simulink model "DAB_OL_loss_cal_2023b"  (R2023b)
settings: Solver=VariableStepAuto  StartTime=0.0  StopTime=0.3  RelTol=1e-3
undefined symbols (not defined in the file): Ion, Lithium, powergui, spspowerguiLib
libraries: spsMeanLib x9, spsMosfetLib x8, spsVoltageMeasurementLib x6, spsCurrentMeasurementLib x4, spsSeriesRLCBranchLib x4, eeGeneralControl x4, spsBatteryLib x1, spsDCVoltageSourceLib x1, spsLinearTransformerLib x1, spsRMSLib x1, simulink x1
settings Model: Creator=Project_Account  LastModifiedBy=saivi
settings ModelReferenceCC: EnableRefExpFcnMdlSchedulingChecks=on
settings ConfigComp: CovBoundaryAbsTol=1.0e-5

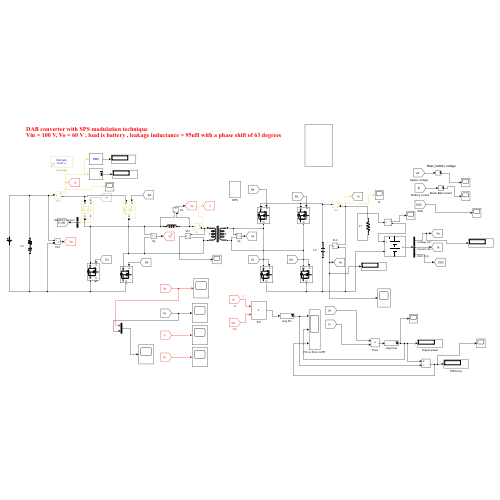
[thumbnail: Simulink's stored preview of the top-level diagram]
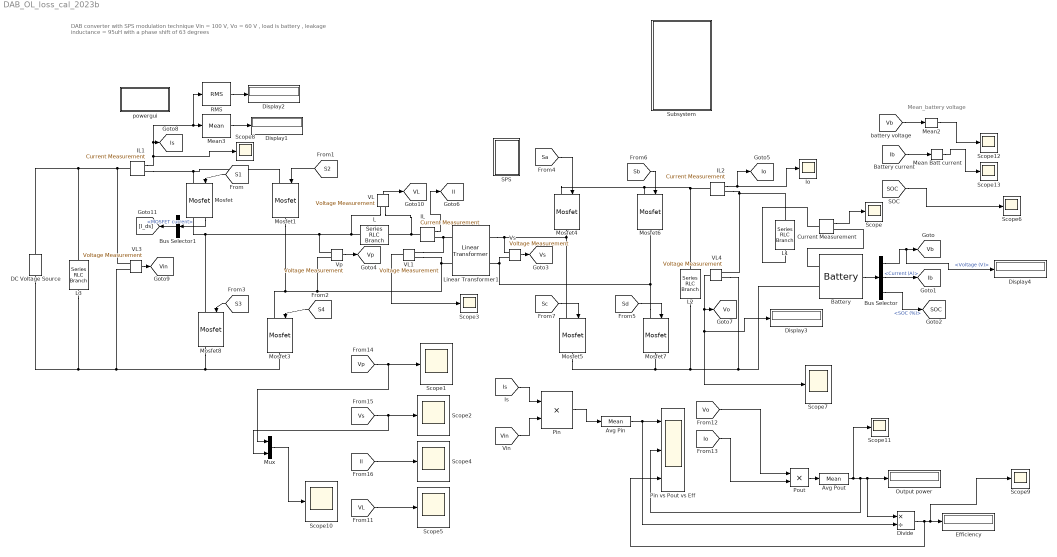
== system DAB_OL_loss_cal_2023b ==
  note: Mean_battery voltage
  note: DAB converter with SPS modulation technique
      | Vin = 100 V, Vo = 60 V , load is battery , leakage inductance = 95uH with a phase shift of 63 degrees
  Avg Pin : spsMeanLib/Mean  Freq=50000  Vinit=0  Ts=1e-7
  Avg Pout : spsMeanLib/Mean  Freq=50000  Vinit=0  Ts=1e-7
  Battery : spsBatteryLib/Battery  BatType=Lithium-Ion  NomV=60  NomQ=120  SOC=60  Batt_Tr=0.1  PresetModel=on  MaxQ=120  MinV=45  FullV=69.8392  Dis_rate=52.1739  R=0.005  Normal_OP=108.5217  expZone="[64.8232      5.89565]"
  Bus Selector : BusSelector  OutputSignals=Voltage (V),Current (A),SOC (%)
  Bus Selector1 : BusSelector  OutputSignals=MOSFET current
  Current Measurement : spsCurrentMeasurementLib/Current Measurement  PhasorSimulation=off  OutputType=Complex  PSBequivalent=0
  DC Voltage Source : spsDCVoltageSourceLib/DC Voltage Source  Amplitude=400  Measurements=None
  Display{1..4} (4 alike) : Display
  Divide : Product  Inputs=*/
  Efficiency : Display
  IL : spsCurrentMeasurementLib/Current Measurement  PhasorSimulation=off  OutputType=Complex  PSBequivalent=0
  IL1 : spsCurrentMeasurementLib/Current Measurement  PhasorSimulation=off  OutputType=Complex  PSBequivalent=0
  IL2 : spsCurrentMeasurementLib/Current Measurement  PhasorSimulation=off  OutputType=Complex  PSBequivalent=0
  Io : Scope
  L : spsSeriesRLCBranchLib/Series RLC Branch  LConnTagsString=__new0  RConnTagsString=__new0  BranchType=L  Resistance=1  Inductance=95e-6  SetiL0=off  InitialCurrent=0  Capacitance=1e-6  Setx0=off  InitialVoltage=0  Measurements=None
  L1 : spsSeriesRLCBranchLib/Series RLC Branch  LConnTagsString=__new0  RConnTagsString=__new0  BranchType=R  Resistance=0.01  Inductance=19.108e-6*2  SetiL0=off  InitialCurrent=0  Capacitance=1000e-6  Setx0=off  InitialVoltage=0  Measurements=None
  L2 : spsSeriesRLCBranchLib/Series RLC Branch  LConnTagsString=__new0  RConnTagsString=__new0  BranchType=C  Resistance=0.8  Inductance=19.108e-6*2  SetiL0=off  InitialCurrent=0  Capacitance=1200e-6  Setx0=off  InitialVoltage=0  Measurements=None
  L3 : spsSeriesRLCBranchLib/Series RLC Branch  LConnTagsString=__new0  RConnTagsString=__new0  BranchType=RC  Resistance=0.8  Inductance=19.108e-6*2  SetiL0=off  InitialCurrent=0  Capacitance=1200e-6  Setx0=off  InitialVoltage=0  Measurements=None
  Linear Transformer1 : spsLinearTransformerLib/Linear Transformer  UNITS=SI  NominalPower=[1500 50000 ]  winding1=[400 0 0]  winding2=[60 0 0]  ThreeWindings=off  winding3=[3.15e+05 0.7938 0.084225]  RmLm=[5000 5866]  Measurements=None  DataType=on
  Mean Batt current : spsMeanLib/Mean  Freq=20000  Vinit=0  Ts=1e-7
  Mean2 : spsMeanLib/Mean  Freq=20000  Vinit=0  Ts=1e-7
  Mean3 : spsMeanLib/Mean  Freq=15000  Vinit=0  Ts=1e-6
  Mosfet : spsMosfetLib/Mosfet  Ron=0.01  Lon=0  Rd=0.01  Vfd=0  IC=0  Rs=1e5  Cs=inf  Measurements=on
  Mosfet{1,3..7} (6 alike) : spsMosfetLib/Mosfet  Ron=0.01  Lon=0  Rd=0.01  Vfd=0  IC=0  Rs=1e5  Cs=inf  Measurements=off
  Mosfet8 : spsMosfetLib/Mosfet  Ron=0.01  Lon=0  Rd=0.01  Vfd=0  IC=0  Rs=1e5  Cs=inf  Measurements=on
  Mux : Mux  Inputs=2
  Output power : Display
  Pin : Product
  "Pin vs Pout vs Eff " : Scope  NumInputPorts=3
  Pout : Product
  RMS : spsRMSLib/RMS  TrueRMS=on  Freq=60  RMSInit=120  Ts=0
  SPS : Subsystem
  Scope{,1..13} (14 alike) : Scope
  Subsystem : Subsystem
  VL{,1,3..4} (4 alike) : spsVoltageMeasurementLib/Voltage Measurement  PhasorSimulation=off  OutputType=Complex  PSBequivalent=0
  Vp : spsVoltageMeasurementLib/Voltage Measurement  PhasorSimulation=off  OutputType=Complex  PSBequivalent=0
  Vs : spsVoltageMeasurementLib/Voltage Measurement  PhasorSimulation=off  OutputType=Complex  PSBequivalent=0
  powergui : Subsystem  Priority=1  AncestorBlock=spspowerguiLib/powergui  InitFcn=powergui( 'InitFcn_Callback' , gcb , 0 , [ ] );  mask(PSB option menu block){SimulationMode=Discrete, SampleTime=1e-7, frequency=60, Iterations=50, frequencyindice=0, Pbase=100e6, ErrMax=1e-4, UnitsV=kV, UnitsW=MW, buscounter=0, FunctionMessages=off, echomessages=off, EnableUseOfTLC=off, CurrentSourceSwitches=off, DisableSnubberDevices=off, DisableRonSwitches=off, DisableVfSwitches=off, DisplayEquations=off, AutomaticDiscreteSolvers=off, SolverType=Tustin/Backward Euler (TBE), Interpol=off, ExternalGateDelay=off, methode=off, Ts=100, x0status=blocks, SPID=on, SwTol=0, HookPort=off, NonlinearTolerance=1e-6, nMaxIteration=1000, ContinueOnMaxIteration=off, RestoreLinks=warning, ResistiveCurrentMeasurement=off, Frange=[0:2:500], Ylog=off, Xlog=on, ShowGrid=off, save=off, variable=ZData, structure=0, ZoomFFT=off, StartTime=0.0, cycles=1, DisplayStyle=1, fundamental=60, FreqAxis=off, MaxFrequency=1000, frequencyindicesteady=1, RmsSteady=1, display=off}
      mask prompts: SimulationMode "Simulation type:"; SampleTime "Sample time (s):"; frequency "Frequency (Hz):"; Iterations "Max iterations"; frequencyindice "Frequency (Hz)"; Pbase "Base power (VA)"; ErrMax "PQ tolerance (pu)"; UnitsV "Voltage units"; UnitsW "Power units"; buscounter "Load flow bus counter"; FunctionMessages "Disable Specialized Power Systems warnings"; echomessages "Display Specialized Power Systems compilation messages"; EnableUseOfTLC "Use TLC file when in Accelerator Simulation Mode and for code generation"; CurrentSourceSwitches "Disable ideal switching"; DisableSnubberDevices "Disable snubbers in switching devices"; DisableRonSwitches "Disable Ron resistances in switching devices"; DisableVfSwitches "Disable forward voltages in switching devices"; DisplayEquations "Display circuit differential equations"; AutomaticDiscreteSolvers "Automatically handle Discrete solver and Advanced tab solver settings of blocks"; SolverType "Discrete solver"; Interpol "Interpolate switching events"; ExternalGateDelay "Use time-stamped gate signals"; methode "Store switching topologies"; Ts "Buffer size (MBytes):"; x0status "Start simulation with initial electrical states from:"; SPID "Use ideal switching devices"; SwTol "Switch tolerance"; HookPort "Allow multiple powergui blocks"; NonlinearTolerance "Solver tolerance"; nMaxIteration "Maximum number of iterations"; ContinueOnMaxIteration "Continue Simulation if maximum number of iterations is reached"; RestoreLinks "Restore disabled links of Simscape Power Systems ST blocks:"; ResistiveCurrentMeasurement "Use non ideal current measurement blocks (1e-4Ohm internal resistance)"; Frange "Frequency Range"; Ylog "Log impedance"; Xlog "log Frequency"; ShowGrid "grid"; save "Save Data To Workspace"; variable "Variable Name"; structure "Structure Name (PSBFFTSCOPE)"; ZoomFFT "ZoomFFT (PSBFFTSCOPE)"; StartTime "Start Time (PSBFFTSCOPE)"; cycles "Cycles (PSBFFTSCOPE)"; DisplayStyle "Display style (PSBFFTSCOPE)"; fundamental "Fundamental (PSBFFTSCOPE)"; FreqAxis "Frequency Axis (PSBFFTSCOPE)"; MaxFrequency "Max Frequency (PSBFFTSCOPE)"; frequencyindicesteady "Frequency indice (STEADYSTATE)"; RmsSteady "RMS display (STEADYSTATE)"; display "Display Results"
      mask help: Set simulation type, simulation parameters, and preferences.
      mask init:
      | dispMessage = '';
      | dispMessage = powergui('MaskInitialization',gcb,SimulationMode,SampleTime);
      settings: PreSaveFcn=powergui( 'PreSaveFcn_Callback' , gcb , [ ] , [ ] );  OpenFcn=sps_rtmsupport('OpenFcn',gcbh)
      mask Help: helpview(psbhelp)
      mask TypeOptions SimulationMode: Continuous | Discrete | Phasor | Discrete phasor
      mask Callback SimulationMode: powergui('SimulationType',[],[],gcb);
      mask TypeOptions UnitsV: V | kV
      mask TypeOptions UnitsW: W | kW | MW
      mask Callback CurrentSourceSwitches: powergui('SimulationType',[],[],gcb);
      mask Callback AutomaticDiscreteSolvers: powergui('SimulationType',[],[],gcb);
      mask TypeOptions SolverType: Tustin/Backward Euler (TBE) | Tustin | Backward Euler
      mask Callback SolverType: powergui('SimulationType',[],[],gcb);
      mask Callback Interpol: powergui('SimulationType',[],[],gcb);
      mask Callback ExternalGateDelay: powergui('SimulationType',[],[],gcb);
      mask Callback methode: powergui('SimulationType',[],[],gcb);
      mask TypeOptions x0status: blocks | steady | zero
      mask TypeOptions RestoreLinks: yes | warning | no
      mask Callback display: sps_rtmsupport('parametereditingmodes',gcbh) % Will be executed last in parameter callbacks to ensure mask enable consistency
      mask DialogControl SolverTab Prompt: Solver
      mask DialogControl AutoSolverNote Prompt: The Simulation type parameter is governed by Simulink. To access the Powergui solver settings, unselect auto (Automatic solver selection) solver in the Simulink solver options.
      mask DialogControl Apps Prompt: Apps
      mask DialogControl StateAnalyzer Prompt: Measurements and States Analyzer
      mask DialogControl StateAnalyzer Callback: powerStates(bdroot(gcb))
      mask DialogControl LineParameterCalculator Prompt: Line Parameter Calculator
      mask DialogControl LineParameterCalculator Callback:
      | close_system(gcb)
      | powerLineParameters
      mask DialogControl CableParameterCalculator Prompt: Cable Parameter Calculator
      mask DialogControl CableParameterCalculator Callback:
      | close_system(gcb)
      | powerCableParameters
      mask DialogControl LineDecoupler Prompt: Line Decoupler
      mask DialogControl LineDecoupler Tooltip: Click to replace selected Distributed Parameters Line blocks with Decoupling Line blocks
      mask DialogControl LineDecoupler Callback:
      | close_system(gcb);
      | DecouplingLineReplace(gcs)
      mask DialogControl LoadFlowAnalyzer Prompt: Load Flow Analyzer
      mask DialogControl LoadFlowAnalyzer Callback:
      | close_system(gcb)
      | powerLoadFlow
      mask DialogControl LoadFlowParameters Prompt: Load Flow Parameters
      mask DialogControl ImpedanceCalculator Prompt: Impedance Calculator
      mask DialogControl ImpedanceCalculator Callback:
      | close_system(gcb);
      | powerImpedance(bdroot(gcs));
      mask DialogControl FFTAnalyzer Prompt: FFT Analyzer
      mask DialogControl FFTAnalyzer Callback:
      | close_system(gcb)
      | power_fftscope(bdroot(gcb),gcb)
      mask DialogControl LinearSystemAnalyzer Prompt: Linear System Analyzer
      mask DialogControl LinearSystemAnalyzer Callback:
      | close_system(gcb)
      | power_ltiview(bdroot(gcb))
      mask DialogControl HysteresisDesigner Prompt: Hysteresis Designer
      mask DialogControl HysteresisDesigner Callback:
      | close_system(gcb)
      | powerHysteresis('hysteresis.mat')
      mask DialogControl BlockCustomizer Prompt: Block Customizer
      mask DialogControl BlockCustomizer Callback:
      | close_system(gcb);
      | power_customize;
      mask DialogControl ReportGenerator Prompt: Report Generator
      mask DialogControl ReportGenerator Callback:
      | close_system(gcb)
      | power_report(bdroot(gcb))
      mask DialogControl obsolete Prompt: ...
      mask DialogControl MachineInitialization Prompt: Machine Initialization
      mask DialogControl MachineInitialization Callback:
      | close_system(gcb)
      | powericon('machineInitTool',bdroot(gcb),gcb)
      mask DialogControl Preferences Prompt: Preferences
      mask DialogControl Solver Prompt: Solver
      mask DialogControl SolverDetails Prompt: Solver details for nonlinear elements
      mask Display: color('blue'),disp(dispMessage)
  tag scope: Ib=global, Il=global, Io=global, Is=global, SOC=global, VL=global, Vb=global, Vin=global, Vo=global, Vp=global, Vs=global
  wires:
  VL1/1 -> Scope3/1
  [S3] -> Mosfet8/1
  Mean2/1 -> Scope12/1
  [Sb] -> Mosfet6/1
  [Ib] -> Mean Batt current/1
  [Vb] -> Mean2/1
  [Sc] -> Mosfet5/1
  VL4/1 -> Scope7/1, Display3/1, [Vo]
  [Vin] -> Pin/2
  [Vo] -> Pout/1
  VL/1 -> [VL]
  IL2/1 -> [Io], Io/1
  [S2] -> Mosfet1/1
  VL3/1 -> [Vin]
  [S4] -> Mosfet3/1
  Vp/1 -> [Vp]
  Mean3/1 -> Display1/1
  IL1/1 -> Scope8/1, RMS/1, Mean3/1, [Is]
  Bus Selector/1 -> Display4/1, [Vb]  "<Voltage (V)>"
  [Sd] -> Mosfet7/1
  RMS/1 -> Display2/1
  [Io] -> Pout/2
  Vs/1 -> [Vs]
  Mean Batt current/1 -> Scope13/1
  [SOC] -> Scope6/1
  [S1] -> Mosfet/1
  [Vp] -> Mux/1, Scope1/1
  Bus Selector/2 -> [Ib]  "<Current (A)>"
  IL/1 -> [Il]
  [Sa] -> Mosfet4/1
  Battery/1 -> Bus Selector/1
  Bus Selector/3 -> [SOC]  "<SOC (%)>"
  Avg Pout/1 -> Scope11/1, "Pin vs Pout vs Eff "/2, Divide/1, Output power/1
  Divide/1 -> "Pin vs Pout vs Eff "/3, Scope9/1, Efficiency/1
  Pout/1 -> Avg Pout/1
  Avg Pin/1 -> Divide/2, "Pin vs Pout vs Eff "/1
  Pin/1 -> Avg Pin/1
  [Is] -> Pin/1
  [Vs] -> Mux/2, Scope2/1
  [VL] -> Scope5/1
  [Il] -> Scope4/1
  Mux/1 -> Scope10/1
  Current Measurement/1 -> Scope/1
  Mosfet/1 -> Bus Selector1/1
  Bus Selector1/1 -> [I_ds]  "<MOSFET current>"
  connections:
  Mosfet7/LConn1 -- Vs/LConn2 -- Linear Transformer1/RConn2 -- Mosfet6/RConn1
  IL/LConn1 -- VL/LConn2 -- L/RConn1
  Linear Transformer1/RConn1 -- Vs/LConn1 -- Mosfet5/LConn1 -- Mosfet4/RConn1
  Vp/LConn2 -- VL1/LConn2 -- Linear Transformer1/LConn2 -- Mosfet3/LConn1 -- Mosfet1/RConn1
  VL1/LConn1 -- Linear Transformer1/LConn1 -- IL/RConn1
  Mosfet3/RConn1 -- Mosfet8/RConn1 -- DC Voltage Source/LConn1 -- L3/RConn1 -- VL3/LConn2
  Mosfet/RConn1 -- Vp/LConn1 -- VL/LConn1 -- L/LConn1 -- Mosfet8/LConn1
  VL3/LConn1 -- IL1/LConn1 -- L3/LConn1 -- DC Voltage Source/RConn1
  Mosfet/LConn1 -- Mosfet1/LConn1 -- IL1/RConn1
  L1/LConn1 -- IL2/RConn1 -- VL4/LConn1
  Mosfet4/LConn1 -- L2/LConn1 -- IL2/LConn1 -- Mosfet6/LConn1
  L2/RConn1 -- Battery/LConn2 -- VL4/LConn2 -- Mosfet7/RConn1 -- Mosfet5/RConn1
  Current Measurement/LConn1 -- L1/RConn1
  Battery/LConn1 -- Current Measurement/RConn1

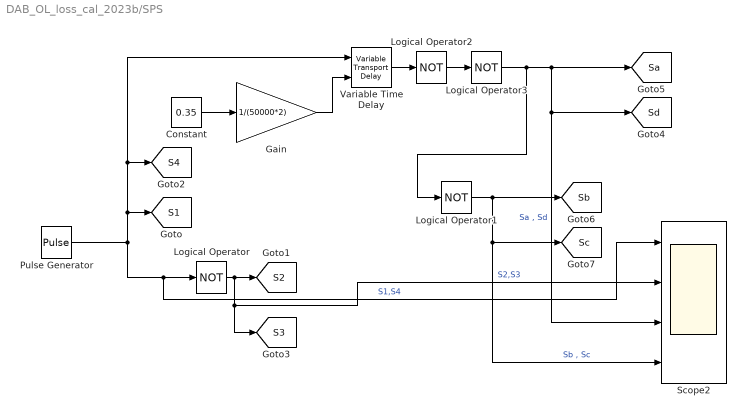
== system DAB_OL_loss_cal_2023b/SPS ==
  Constant : Constant  Value=0.35
  Gain : Gain  Gain=1/(50000*2)
  Logical Operator{,1..3} (4 alike) : Logic  Operator=NOT  AllPortsSameDT=off  OutDataTypeStr=boolean
  Pulse Generator : DiscretePulseGenerator  PulseType=Time based  Period=1/50000  PulseWidth=50
  Scope2 : Scope  NumInputPorts=4
  Variable Time Delay : VariableTransportDelay  MaximumDelay=10
  tag scope: S1=global, S2=global, S3=global, S4=global, Sa=global, Sb=global, Sc=global, Sd=global
  wires:
  Variable Time Delay/1 -> Logical Operator2/1
  Logical Operator1/1 -> Scope2/4, [Sc], [Sb]  "Sb , Sc"
  Pulse Generator/1 -> Variable Time Delay/1, [S4], [S1], Scope2/1, Logical Operator/1  "S1,S4"
  Logical Operator/1 -> [S3], Scope2/2, [S2]  "S2,S3"
  Gain/1 -> Variable Time Delay/2
  Constant/1 -> Gain/1
  Logical Operator2/1 -> Logical Operator3/1
  Logical Operator3/1 -> Logical Operator1/1, [Sa], Scope2/3, [Sd]  "Sa , Sd"

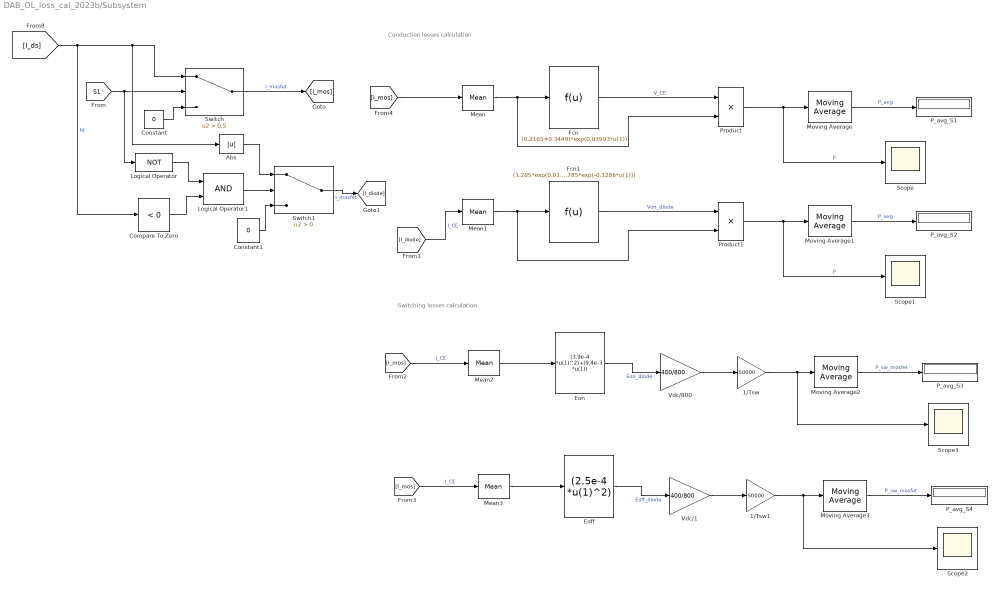
== system DAB_OL_loss_cal_2023b/Subsystem ==
  note: Switching losses calculation
  note: Conduction losses calculation
  1/Tsw : Gain  Gain=50000
  1/Tsw1 : Gain  Gain=50000
  Abs : Abs  SaturateOnIntegerOverflow=off
  Compare To Zero : simulink/Logic and Bit Operations/Compare To Zero  relop=<  OutDataTypeStr=boolean
  Constant : Constant  Value=0
  Constant1 : Constant  Value=0
  Eoff : Fcn  Expr=(2.5e-4 *u(1)^2)
  Eon : Fcn  Expr=(3.9e-4 *u(1)^2)+(9.4e-3 *u(1))
  Fcn : Fcn  Expr=(0.2165+0.3449)*exp(0.03993*u(1))
  Fcn1 : Fcn  Expr=(1.285*exp(0.0139*u(1)))-(0.785*exp(-0.1286*u(1)))
  Logical Operator : Logic  Operator=NOT  AllPortsSameDT=off  OutDataTypeStr=boolean
  Logical Operator1 : Logic  AllPortsSameDT=off  OutDataTypeStr=boolean
  Mean{,1..3} (4 alike) : spsMeanLib/Mean  Freq=60  Vinit=0  Ts=0
  Moving Average{,1..3} (4 alike) : eeGeneralControl/Moving Average  VariantControl=Variant1  LabelModeActiveChoice=Discrete  f=60  x0=0  BufferSize=8192  Ts=-1
      settings: LibrarySourceBlock=ee_sl_lib/General Control/Moving Average
  P_avg_S{1..4} (4 alike) : Display
  Product : Product
  Product1 : Product
  Scope{,1..3} (4 alike) : Scope
  Switch : Switch  Criteria=u2 > Threshold  Threshold=0.5  SaturateOnIntegerOverflow=off  InputSameDT=off
  Switch1 : Switch  Criteria=u2 > Threshold  SaturateOnIntegerOverflow=off  InputSameDT=off
  Vdc/1 : Gain  Gain=400/800
  Vdc/800 : Gain  Gain=400/800
  wires:
  Fcn/1 -> Product/1  "V_CE"
  Product/1 -> Scope/1, Moving Average/1  "P"
  Moving Average/1 -> P_avg_S1/1  "P_avg"
  Mean/1 -> Product/2, Fcn/1
  Product1/1 -> Scope1/1, Moving Average1/1  "P"
  [I_diode] -> Mean1/1  "I_CE"
  Mean1/1 -> Product1/2, Fcn1/1
  Moving Average1/1 -> P_avg_S2/1  "P_avg"
  Fcn1/1 -> Product1/1  "Von_diode"
  Moving Average2/1 -> P_avg_S3/1  "P_sw_mosfet"
  Mean2/1 -> Eon/1
  [I_mos] -> Mean2/1  "I_CE"
  Eon/1 -> Vdc/800/1  "Eon_diode"
  Vdc/800/1 -> 1/Tsw/1
  1/Tsw/1 -> Scope3/1, Moving Average2/1
  [I_mos] -> Mean3/1  "I_CE"
  1/Tsw1/1 -> Scope2/1, Moving Average3/1
  Mean3/1 -> Eoff/1
  Vdc/1/1 -> 1/Tsw1/1
  Moving Average3/1 -> P_avg_S4/1  "P_sw_mosfet"
  Eoff/1 -> Vdc/1/1  "Eoff_diode"
  [I_ds] -> Compare To Zero/1, Abs/1, Switch/1  "Id"
  [S1] -> Switch/2, Logical Operator/1
  Constant/1 -> Switch/3
  Switch/1 -> [I_mos]  "I_mosfet"
  [I_mos] -> Mean/1
  Logical Operator/1 -> Logical Operator1/1
  Compare To Zero/1 -> Logical Operator1/2
  Logical Operator1/1 -> Switch1/2
  Abs/1 -> Switch1/1
  Constant1/1 -> Switch1/3
  Switch1/1 -> [I_diode]  "I_mosfet"

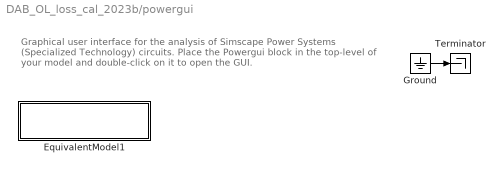
== system DAB_OL_loss_cal_2023b/powergui ==
  note: Graphical user interface for the analysis of
      | Simscape Power Systems (Specialized Technology) circuits.
      | Place the Powergui block in the top-level of your model and double-click
      | on it to open the GUI.
  EquivalentModel1 : Subsystem
      mask init:
      | S  = GetDataForEquivalentModel('Discrete',gcbh);
      mask Display:
      | color('red')
      | disp('EQUIVALENT CIRCUIT\nDiscrete')
  Ground : Ground
  Terminator : Terminator
  wires:
  Ground/1 -> Terminator/1

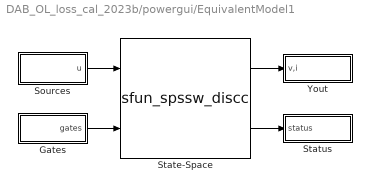
== system DAB_OL_loss_cal_2023b/powergui/EquivalentModel1 ==
  Gates : Subsystem
  Sources : Subsystem
  State-Space : S-Function  FunctionName=sfun_spssw_discc  Parameters=S.Ts,S.A, S.B, S.C, S.D, S.x0, S.EnableUseOfTLC,S.SwitchResistance ,S.SwitchType, S.SwitchGateInitialValue, S.OutputsToResetToZero, S.TBEON,S.SaveMatrices,S.BufferSize  SFunctionDeploymentMode=off  EnableBusSupport=off
  Status : Subsystem
  Yout : Subsystem
  wires:
  Gates/1(gates) -> State-Space/2
  Sources/1(u) -> State-Space/1
  State-Space/2 -> Status/1(status)
  State-Space/1 -> Yout/1(v,i)

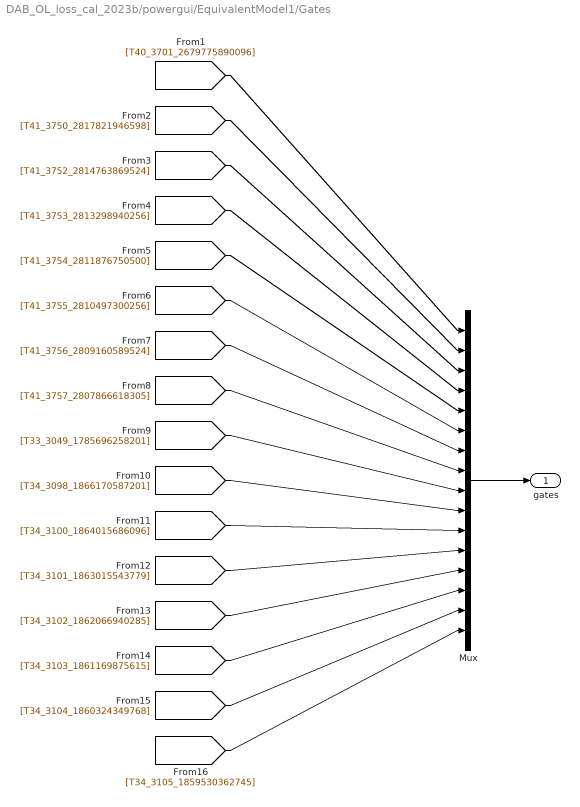
== system DAB_OL_loss_cal_2023b/powergui/EquivalentModel1/Gates ==
  Mux : Mux  Inputs=[1 1 1 1 1 1 1 1 1 1 1 1 1 1 1 1]
  gates : Outport  VectorParamsAs1DForOutWhenUnconnected=off
  wires:
  Mux/1 -> gates/1
  [T40_3701_2679775890096] -> Mux/1
  [T41_3750_2817821946598] -> Mux/2
  [T41_3752_2814763869524] -> Mux/3
  [T41_3753_2813298940256] -> Mux/4
  [T41_3754_2811876750500] -> Mux/5
  [T41_3755_2810497300256] -> Mux/6
  [T41_3756_2809160589524] -> Mux/7
  [T41_3757_2807866618305] -> Mux/8
  [T33_3049_1785696258201] -> Mux/9
  [T34_3098_1866170587201] -> Mux/10
  [T34_3100_1864015686096] -> Mux/11
  [T34_3101_1863015543779] -> Mux/12
  [T34_3102_1862066940285] -> Mux/13
  [T34_3103_1861169875615] -> Mux/14
  [T34_3104_1860324349768] -> Mux/15
  [T34_3105_1859530362745] -> Mux/16

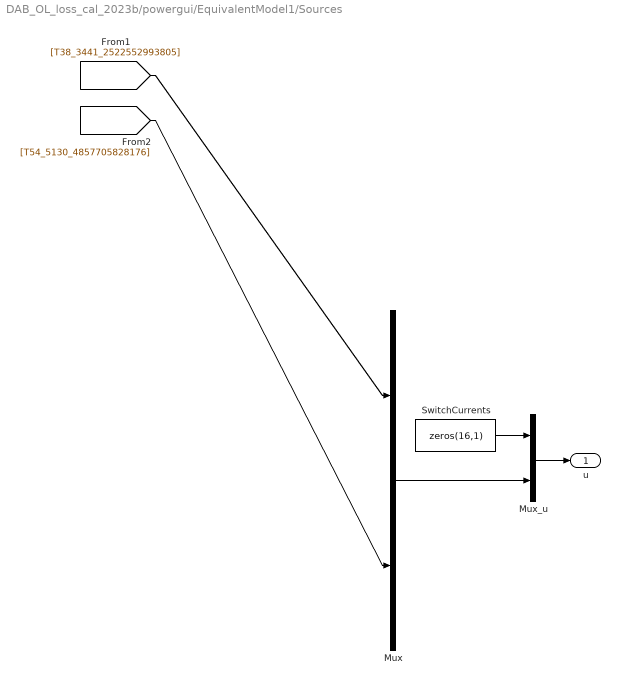
== system DAB_OL_loss_cal_2023b/powergui/EquivalentModel1/Sources ==
  Mux : Mux  Inputs=[1 1]
  Mux_u : Mux  Inputs=[16 2]
  SwitchCurrents : Constant  Value=zeros(16,1)
  u : Outport  VectorParamsAs1DForOutWhenUnconnected=off
  wires:
  Mux_u/1 -> u/1
  SwitchCurrents/1 -> Mux_u/1
  Mux/1 -> Mux_u/2
  [T38_3441_2522552993805] -> Mux/1
  [T54_5130_4857705828176] -> Mux/2

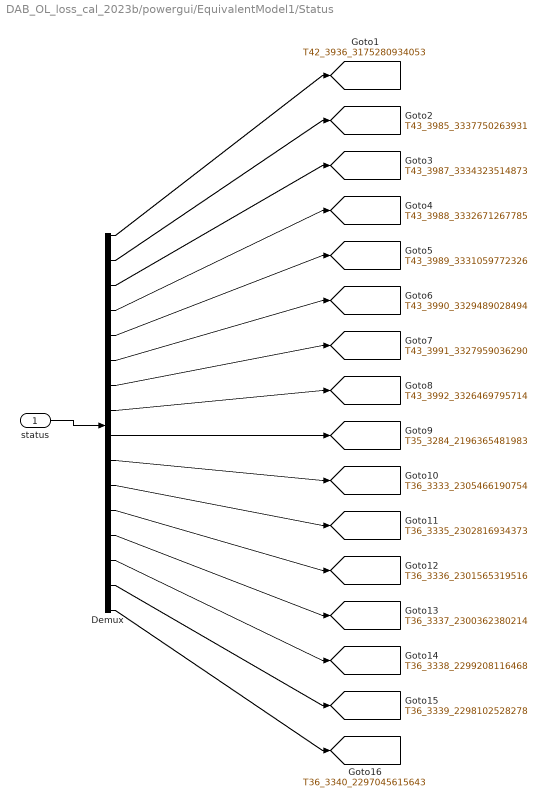
== system DAB_OL_loss_cal_2023b/powergui/EquivalentModel1/Status ==
  status : Inport
  Demux : Demux  Outputs=[1 1 1 1 1 1 1 1 1 1 1 1 1 1 1 1]
  tag scope: T35_3284_2196365481983=global, T36_3333_2305466190754=global, T36_3335_2302816934373=global, T36_3336_2301565319516=global, T36_3337_2300362380214=global, T36_3338_2299208116468=global, T36_3339_2298102528278=global, T36_3340_2297045615643=global, T42_3936_3175280934053=global, T43_3985_3337750263931=global, T43_3987_3334323514873=global, T43_3988_3332671267785=global, T43_3989_3331059772326=global, T43_3990_3329489028494=global, T43_3991_3327959036290=global, T43_3992_3326469795714=global
  wires:
  status/1 -> Demux/1
  Demux/1 -> [T42_3936_3175280934053]
  Demux/2 -> [T43_3985_3337750263931]
  Demux/3 -> [T43_3987_3334323514873]
  Demux/4 -> [T43_3988_3332671267785]
  Demux/5 -> [T43_3989_3331059772326]
  Demux/6 -> [T43_3990_3329489028494]
  Demux/7 -> [T43_3991_3327959036290]
  Demux/8 -> [T43_3992_3326469795714]
  Demux/9 -> [T35_3284_2196365481983]
  Demux/10 -> [T36_3333_2305466190754]
  Demux/11 -> [T36_3335_2302816934373]
  Demux/12 -> [T36_3336_2301565319516]
  Demux/13 -> [T36_3337_2300362380214]
  Demux/14 -> [T36_3338_2299208116468]
  Demux/15 -> [T36_3339_2298102528278]
  Demux/16 -> [T36_3340_2297045615643]

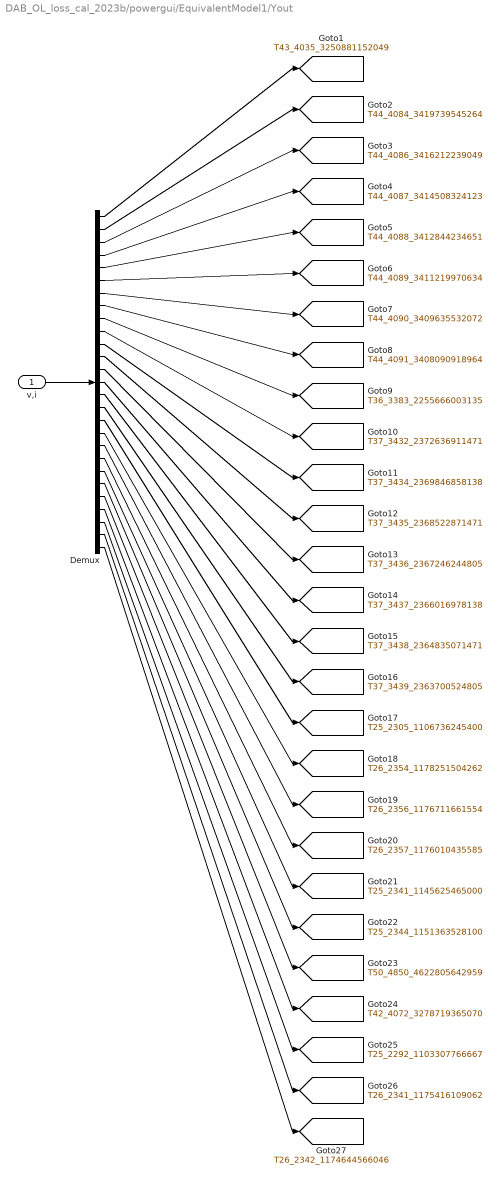
== system DAB_OL_loss_cal_2023b/powergui/EquivalentModel1/Yout ==
  v,i : Inport
  Demux : Demux  Outputs=[1 1 1 1 1 1 1 1 1 1 1 1 1 1 1 1 1 1 1 1 1 1 1 1 1 1 1]
  tag scope: T25_2292_1103307766667=global, T25_2305_1106736245400=global, T25_2341_1145625465000=global, T25_2344_1151363528100=global, T26_2341_1175416109062=global, T26_2342_1174644566046=global, T26_2354_1178251504262=global, T26_2356_1176711661554=global, T26_2357_1176010435585=global, T36_3383_2255666003135=global, T37_3432_2372636911471=global, T37_3434_2369846858138=global, T37_3435_2368522871471=global, T37_3436_2367246244805=global, T37_3437_2366016978138=global, T37_3438_2364835071471=global, T37_3439_2363700524805=global, T42_4072_3278719365070=global, T43_4035_3250881152049=global, T44_4084_3419739545264=global, T44_4086_3416212239049=global, T44_4087_3414508324123=global, T44_4088_3412844234651=global, T44_4089_3411219970634=global, T44_4090_3409635532072=global, T44_4091_3408090918964=global, T50_4850_4622805642959=global
  wires:
  v,i/1 -> Demux/1
  Demux/1 -> [T43_4035_3250881152049]
  Demux/2 -> [T44_4084_3419739545264]
  Demux/3 -> [T44_4086_3416212239049]
  Demux/4 -> [T44_4087_3414508324123]
  Demux/5 -> [T44_4088_3412844234651]
  Demux/6 -> [T44_4089_3411219970634]
  Demux/7 -> [T44_4090_3409635532072]
  Demux/8 -> [T44_4091_3408090918964]
  Demux/9 -> [T36_3383_2255666003135]
  Demux/10 -> [T37_3432_2372636911471]
  Demux/11 -> [T37_3434_2369846858138]
  Demux/12 -> [T37_3435_2368522871471]
  Demux/13 -> [T37_3436_2367246244805]
  Demux/14 -> [T37_3437_2366016978138]
  Demux/15 -> [T37_3438_2364835071471]
  Demux/16 -> [T37_3439_2363700524805]
  Demux/17 -> [T25_2305_1106736245400]
  Demux/18 -> [T26_2354_1178251504262]
  Demux/19 -> [T26_2356_1176711661554]
  Demux/20 -> [T26_2357_1176010435585]
  Demux/21 -> [T25_2341_1145625465000]
  Demux/22 -> [T25_2344_1151363528100]
  Demux/23 -> [T50_4850_4622805642959]
  Demux/24 -> [T42_4072_3278719365070]
  Demux/25 -> [T25_2292_1103307766667]
  Demux/26 -> [T26_2341_1175416109062]
  Demux/27 -> [T26_2342_1174644566046]
